simulink library "carnot"  (R2018b)
settings: Solver=VariableStepAuto  StartTime=0.0  StopTime=10.0  RelTol=1e-3
undefined symbols (not defined in the file or in its folder): A, A_earth, acol, Acol, ActPower1, ActPower2, ActPower3, Ad, Ad0, Ar, Au, Au0, Azimuth_Angle, B, Bd, Bd0, Br, Bu, Bu0, C, c1, c2, c3, c33, c4, c5, c6, CarnotCallbacks_Density, CarnotCallbacks_Enthalpy, CarnotCallbacks_Enthalpy2Temperature, CarnotCallbacks_Entropy, CarnotCallbacks_Evaporation_Enthalpy, CarnotCallbacks_GlobalMessageLevel, CarnotCallbacks_Grashof, CarnotCallbacks_Heat_Capacity, CarnotCallbacks_Kinematic_Viscosity, CarnotCallbacks_PMV_PPD, CarnotCallbacks_Prandtl, CarnotCallbacks_Saturation_Property, CarnotCallbacks_Saturation_Temperature, CarnotCallbacks_Saturation_Value_Water, CarnotCallbacks_Specific_Volume, CarnotCallbacks_Thermal_Conductivity, CarnotCallbacks_Vapour_Content, CarnotCallbacks_Vapour_Pressure, Cd, Cdl, Cr, Cu, Davies, Dd, DE_TRY2010_04_averageYear, delta_grd, density, DiameterLastPiece, dl, DPConstant, DPLinear, DPQuadratic, Dr ... (+59)
libraries: $bdroot x429, simulink x36, simulink_extras x12
(part 8 of 22)

== system carnot/Load/Houses ==
  House_simple : Subsystem  mask(House simple){tini=20, dtroom=inf, Tmeaninside=23.8, deltathetai=3.8, Tmeanoutside=11, deltathetae=9.3, tshift=319*3600, PathName=fullfile(path_carnot('libsl'), 'Load', 'Houses', 'House_simple', 'parameter_set'), FileName='Default_SimpleHouseISOgm.mat', userPath=off, userParam=off, Ahabit=140, Hroom=2.5, slabwidth=10, slablength=7, dwall=0.4, UAwall=100, capa=500000, utot=0.183, gammat=0, cond_ground=2, cp_ground=800, rho_ground=2500, Awindow=[12 4 3 4], AziWin=[0 90 -180 -90], Uwindow=[2 2 2 2], Gwindow=[0.5 0.5 0.5 0.5], alpha=10, H=1.2, W=1, Nwin=4, Ventilationrate=0.4, Heatrecovery=0, pnom=10000, dtnom=49.83, expo=1.3, mcap=10*4812, lin=100, qua=100}
      mask prompts: tini "Initial temperature in °C"; dtroom "Max. change of room temperature in K (standard value is 'inf')"; Tmeaninside "Mean inside temperature over one year [°C]"; deltathetai "Amplitude of monthly mean inside temperature over the year [K]"; Tmeanoutside "Mean outside temperature over one year [°C]"; deltathetae "Amplitude of monthly mean outside temperature over the year [K]"; tshift "Time shift where outside temperature sine-curve shows a mimimum [s]"; PathName "Path"; FileName "Parameter set"; userPath "Edit path and name of parameter set"; userParam "User defined parameters"; Ahabit "Heated living surface in m²"; Hroom "Height of rooms in m"; slabwidth "Width of slab in m"; slablength "Length of slab in m"; dwall "Average thickness of walls inlcuding insulation [m]"; UAwall "Total heat transfer to ambient (walls/roof) in W/K"; capa "Thermal capactiy per surface in J/m²/K"; utot "Total heat transfer of slab to ground [W/m²/K]"; gammat "linear thermal transmittance associated with wall/floor junctions [W/mK]"; cond_ground "conductivity of ground [W/(m*K)]"; cp_ground "capacity of ground [J/(kg*K)]"; rho_ground "density of ground [kg/m^3]"; Awindow "Surface of 4 windows in m² (vector)"; AziWin "Orientation of the 4 windows (south 0, east -90,west 90)"; Uwindow "Heat loss coefficient 4 windows in W/m²/K [vector]"; Gwindow "Light transmittance 4 windows (0..1) * (1 - frame_part) [vector]"; alpha "Maximal opening angle in °"; H "Height of window opening in m"; W "Width of window opening in m"; Nwin "Number of windows for ventilation"; Ventilationrate "Ventilation rate in 1/h"; Heatrecovery "Heat recovery (0..1)"; pnom "Qdot_nom: nominal power in W"; dtnom "Tdiff_nom: nominal temperature difference in K"; expo "Radiator exponent (> 0)"; mcap "mass * capacity in J/K"; lin "l : linear pressure drop Pa/(kg/s)"; qua "q : quadratic pressure drop Pa/(kg/s)²"
      mask help:
      | Simple model of a house with one thermal node. The geometry is a box with a flat roof and 4 windows (see House_OneNodeModel). The heat transfer to the ground is modeled by HeatTransfer2Ground_ISO13370. The heating system is the Radiator model. The ventilation an heat recovery uses the Ventilation model. Resident data like internal gains, window opening and shading are defined by the Resident Data Bus RDB.
      |
      | Max. change of room temperatue: Set parameter to 0 K to calculate idealized heating behaviour. The power balance (Qdot_all) is the theoretical heating demand (see example_House_Ideal.slx).
      mask init:
      | [ok, param] = CarnotCallbacks_HouseSimple('SetParameters',gcbh,PathName,FileName);
      mask Help: web(fullfile(path_carnot('help'),'houseSimple.html'),'-helpbrowser')
      mask TypeOptions tini: House_OneNodeModel/tini | Radiator/tini
      mask TypeOptions dtroom: House_OneNodeModel/dtroom
      mask TypeOptions Tmeaninside: HeatTransfer2Ground_ISO13370/Tmeaninside
      mask TypeOptions deltathetai: HeatTransfer2Ground_ISO13370/deltathetai
      mask TypeOptions Tmeanoutside: HeatTransfer2Ground_ISO13370/Tmeanoutside
      mask TypeOptions deltathetae: HeatTransfer2Ground_ISO13370/deltathetae
      mask TypeOptions tshift: HeatTransfer2Ground_ISO13370/tshift
      mask Callback userPath: [ok, param] = CarnotCallbacks_HouseSimple('UserEdit',gcbh);
      mask Callback userParam: [ok, param] = CarnotCallbacks_HouseSimple('UserEdit',gcbh);
      mask TypeOptions Ahabit: House_OneNodeModel/A | Ventilation/Ahabit | Ahabit/Value
      mask TypeOptions Hroom: Simple_House_ISO_GroundModel/Hroom | Ventilation/Hroom
      mask TypeOptions slabwidth: HeatTransfer2Ground_ISO13370/slabwidth
      mask TypeOptions slablength: HeatTransfer2Ground_ISO13370/slablength
      mask TypeOptions dwall: HeatTransfer2Ground_ISO13370/dwall
      mask TypeOptions UAwall: House_OneNodeModel/UAout
      mask TypeOptions capa: House_OneNodeModel/capa
      mask TypeOptions utot: HeatTransfer2Ground_ISO13370/utot
      mask TypeOptions gammat: HeatTransfer2Ground_ISO13370/gammat
      mask TypeOptions cond_ground: HeatTransfer2Ground_ISO13370/cond_ground
      mask TypeOptions cp_ground: HeatTransfer2Ground_ISO13370/cp_ground
      mask TypeOptions rho_ground: HeatTransfer2Ground_ISO13370/rho_ground
      mask TypeOptions Awindow: House_OneNodeModel/Awin
      mask TypeOptions AziWin: House_OneNodeModel/AziWin
      mask TypeOptions Uwindow: House_OneNodeModel/Uwin
      mask TypeOptions Gwindow: House_OneNodeModel/Gwin
      mask TypeOptions alpha: Ventilation/alpha
      mask TypeOptions H: Ventilation/H
      mask TypeOptions W: Ventilation/W
      mask TypeOptions Nwin: Ventilation/Nwin
      mask TypeOptions Ventilationrate: Ventilation/vent
      mask TypeOptions Heatrecovery: Ventilation/rec
      mask TypeOptions pnom: Radiator/pnom
      mask TypeOptions dtnom: Radiator/dtnom
      mask TypeOptions expo: Radiator/expo
      mask TypeOptions mcap: Radiator/mcap
      mask TypeOptions lin: Radiator/lin
      mask TypeOptions qua: Radiator/qua
      mask DialogControl Container10 Prompt: Calculation
      mask DialogControl ParameterGroupFile Prompt: Picking a parameter set
      mask DialogControl Control1 Prompt: Carnot public data
      mask DialogControl Control1 Callback: [ok, file] = CarnotCallbacks_HouseSimple('GetFilename',gcbh, 'public');
      mask DialogControl Control3 Prompt: Carnot internal data
      mask DialogControl Control3 Callback: [ok, file] = CarnotCallbacks_HouseSimple('GetFilename',gcbh, 'internal');
      mask DialogControl Control4 Prompt: Selected path
      mask DialogControl Control4 Callback: [ok, file] = CarnotCallbacks_HouseSimple('GetFilename',gcbh, 'selected');
      mask DialogControl Container5 Prompt: House
      mask DialogControl Container13 Prompt: Ground
      mask DialogControl Container8 Prompt: Windows
      mask DialogControl Container9 Prompt: HVAC
      mask DialogControl Control5 Prompt: Save in Carnot internal data
      mask DialogControl Control5 Callback: [ok, param] = CarnotCallbacks_HouseSimple('SaveFilename',gcbh, 'internal','SH');
      mask DialogControl Control6 Prompt: Save in selected path
      mask DialogControl Control6 Callback: [ok, param] = CarnotCallbacks_HouseSimple('SaveFilename',gcbh, 'selected','SH');
      mask Display:
      | % user defined picture file
      | picfile = fullfile(path_carnot('intlibsl'), ...
      |         'Load','Houses','Simple_House_ISOgm_CONF','parameter_set', ...
      |         'Simple_House_ISOgm_CONF.jpg');
      | 
      | % show internal picture if defined
      | if ~BlockIsInCarnotLibrary ...      % if not located in library any more
      |         && exist(picfile,'file')    % AND picfile is present
      |     image(imread(picfile), [0.15 0.1 0.7 0.8])
      |     set_param(gcb, 'BackgroundColor', 'White')
      | else
      |     % show public picture
      |     plot([10,10,90,90,10]/120+0.1, [0,50,50,0,0]/100+0.1,...
      |          [100,60,40,0]/120+0.1,    [40,80,80,40]/100+0.1,...
      |          [20,34,34,20,20]/120+0.1, [40,40,20,20,40]/100+0.1,...
      |          [60,60,40,40]/120+0.1,    [0,40,40,0]/100+0.1,...
      |          [65,80,80,65,65]/120+0.1, [40,40,20,20,40]/100+0.1,...
      |          [47,54,54,47,47]/120+0.1, [35,35,4,4,35]/100+0.1,...
      |          [45,41]/120+0.1,          [20,20]/100+0.1)
      |      set_param(gcb, 'BackgroundColor', 'Orange')
      | end
  Resident_Data : Subsystem  mask(Resident Task){CalcAirComp=on}
      mask prompts: CalcAirComp "Calculate the composition of room air (H2O, CO2, VOC)"
      mask help:
      | Create the Resident Data Bus.
      | Qdot_internal : internal gains in the building in W
      | Sunshade : shading of the windows [0..1]
      | 	0 : no shading
      | 	1 : complete shading
      | OpenWindow : open the windows [0..1]
      | 	0 : closed
      | 	1 : completely opened
      | Massflow_CO2 : massflow of CO2 generated by internal sources in kg/s
      | Massflow_H2O : massflow of HO generated by internal sources in kg/s
      | Massflow_VOC : massflow of VOCs generated by internal sources in kg/s
      mask TypeOptions CalcAirComp: CalculateAirComposition/CalcAirComp
      mask Display:
      | plot(-20,-20,100,100,[30,70,70,30,30],[80,80,30,30,80],...
      |     [65,60,40,35],[30,40,40,30],...
      |     [53,53,56,56,50,44,44,47,47],...
      |     [40,45,49,60,65,60,50,45,40],...
      |     [57,50,44],[40,34,40],...
      |     [52,53],[55,55],[47,48],[55,55],...
      |     [56,53,47,44],[51,60,60,51],[52,50,48],[49,48,49])
  Resident_Task44 : Subsystem  mask(Resident Task){period=24*3600, rep_seq_te=[0 1 6 7 8 9 11 12 13 18 19 20 22 23]*3600, rep_seq_de=[1 5 1 1 1 2 1 1 4 2 1 2 1 1]*3600, rep_seq_ye=[105 55 392.5 457.5 420 55 250 55 120 170 615 420 442.5 355], rep_seq_to=[0 6 7 8 9 11 12 13 14 15 17 18 20 21 22]*3600, rep_seq_do=[6 1 1 1 2 1 1 1 1 2 1 2 1 1 2]*3600, rep_seq_yo=[4 2 3 2 0 1 3 2 1 0 1 2 4 3 4]*60, Topen=24, Tclose=23, TrAboveTa=2, TaTooCold=12, timeFIR=24, TaIni=12, starttime=8, stoptime=22, TroomShadeOn=23.8, TroomShadeOff=22.8, SolarShadeOn=300, SolarShadeOff=200, max_shade=1, CalcAirComp=off, mdotCO2=0, mdotH2O=0, mdotVOC=0}
      mask prompts: period "Time period in s"; rep_seq_te "Time values in s"; rep_seq_de "Duration in s"; rep_seq_ye "Internal gains due to electricity consumption in W"; rep_seq_to "Time values in s"; rep_seq_do "Duration in s"; rep_seq_yo "Internal gain due to persons in W"; Topen "Open window if Troom is above [°C]"; Tclose "Close window if Troom is below [°C]"; TrAboveTa "Open window if Troom is above Tamb [K]"; TaTooCold "Close window if average Tamb is below [°C]"; timeFIR "Average time for Tamb in h (only integer values)"; TaIni "Initial value for Tamb in °C"; starttime "Start time in the morning [h]"; stoptime "Stop time in the evening [h]"; TroomShadeOn "Room temperature to switch shading on in °C"; TroomShadeOff "Room temperature to switch shading off in °C"; SolarShadeOn "Solar radiation to switch shading on in W/m²"; SolarShadeOff "Solar radiation to switch shading off in W/m²"; max_shade "Maximum value for Sunshade"; CalcAirComp "Calculate the composition of room air (H2O, CO2, VOC)"; mdotCO2 "Massflow CO2 in kg/s"; mdotH2O "Massflow H2O in kg/s"; mdotVOC "Massflow VOC in kg/s"
      mask help: Create the Resident Data Bus for boundary conditions of Task 44.
      mask TypeOptions period: Electric_Gains_Profile/period | Occupation_Profile/period
      mask TypeOptions rep_seq_te: Electric_Gains_Profile/rep_seq_t
      mask TypeOptions rep_seq_de: Electric_Gains_Profile/rep_seq_d
      mask TypeOptions rep_seq_ye: Electric_Gains_Profile/rep_seq_y
      mask TypeOptions rep_seq_to: Occupation_Profile/rep_seq_t
      mask TypeOptions rep_seq_do: Occupation_Profile/rep_seq_d
      mask TypeOptions rep_seq_yo: Occupation_Profile/rep_seq_y
      mask TypeOptions Topen: Window_Control/Topen
      mask TypeOptions Tclose: Window_Control/Tclose
      mask TypeOptions TrAboveTa: Window_Control/TrAboveTa
      mask TypeOptions TaTooCold: Window_Control/TaTooCold
      mask TypeOptions timeFIR: Window_Control/timeFIR
      mask TypeOptions TaIni: Window_Control/TaIni
      mask TypeOptions starttime: Window_Control/starttime
      mask TypeOptions stoptime: Window_Control/stoptime
      mask TypeOptions TroomShadeOn: Shading_Control/TroomShadeOn
      mask TypeOptions TroomShadeOff: Shading_Control/TroomShadeOff
      mask TypeOptions SolarShadeOn: Shading_Control/SolarShadeOn
      mask TypeOptions SolarShadeOff: Shading_Control/SolarShadeOff
      mask TypeOptions max_shade: Shading_Control/max_shade
      mask TypeOptions CalcAirComp: CalculateAirComposition/CalcAirComp
      mask TypeOptions mdotCO2: Massflow_CO2/Value
      mask TypeOptions mdotH2O: Massflow_H2O/Value
      mask TypeOptions mdotVOC: Massflow_VOC/Value
      mask DialogControl Container5 Prompt: Internal gain
      mask DialogControl Container6 Prompt: Electric gains profile
      mask DialogControl Container7 Prompt: Occupation profile
      mask DialogControl Container8 Prompt: Windows
      mask DialogControl Container10 Prompt: Ventilation cooling
      mask DialogControl Container9 Prompt: Shading
      mask DialogControl Container11 Prompt: Emissions
      mask Display:
      | plot(0,0,100,100,[30,70,70,30,30],[80,80,30,30,80],...
      |     [65,60,40,35],[30,40,40,30],...
      |     [53,53,56,56,50,44,44,47,47],...
      |     [40,45,49,60,65,60,50,45,40],...
      |     [57,50,44],[40,34,40],...
      |     [52,53],[55,55],[47,48],[55,55],...
      |     [56,53,47,44],[51,60,60,51],[52,50,48],[49,48,49])
      | disp('\n\n\n\n\nTASK 44')
  Room_Floor_Heating : Subsystem  mask(room){t0=20, temp_neighbour=20}
      mask prompts: t0 "start temperature of rooms in °C"; temp_neighbour "temperature of rooms above and below in °C"
      mask help:
      | The block models of a heat transfer characteristic of two neighbour rooms.
      | Use "look under mask" to set up the models parameters (initial conditions,
      | floors and wall characteristics...)
      mask init:
      | AIV_neighbour = [0 temp_neighbour temp_neighbour 0 0 0 0 0 0];
      | zonefloordist2grnd = 0;
      mask Help: web(fullfile(path_carnot('help'),'Room_Floor_Heating.html'),'-helpbrowser')
      mask Display: plot(0,0,100,100,[30,30,60,60,30],[20,50,50,20,20],[47,47,56,56,47],[40,30,30,40,40],[42,42,34,34],[20,40,40,20],[62,45,28],[48,70,48])
  Room_Radiator : Subsystem  mask(room){t0=20, temp_neighbour=20}
      mask prompts: t0 "start temperature of rooms in °C"; temp_neighbour "temperature of rooms above and below in °C"
      mask help:
      | The block models of a heat transfer characteristic of two neighbour rooms.
      | Use "look under mask" to set up the models parameters (initial conditions,
      | floors and wall characteristics...)
      mask init:
      | AIV_neighbour = [0 temp_neighbour temp_neighbour 0 0 0 0 0 0];
      | zonefloordist2grnd = 0;
      mask Help: web(fullfile(path_carnot('help'),'Room_Radiator.html'),'-helpbrowser')
      mask Display: plot(0,0,100,100,[30,30,60,60,30],[20,50,50,20,20],[47,47,56,56,47],[40,30,30,40,40],[42,42,34,34],[20,40,40,20],[62,45,28],[48,70,48])

== system carnot/Outputs/AIV_selector ==
  "[AIV]" : Inport
  Selector : Selector  InputPortWidth=9  IndexOptions=Index vector (dialog)  Indices=v  OutputSizes=1
  "[AIV]s" : Outport
  wires:
  Selector/1 -> "[AIV]s"/1
  "[AIV]"/1 -> Selector/1

== system carnot/Outputs/Display_THB1 ==
  THB_yellow : Inport
  Selector : Selector  InputPortWidth=20  IndexOptions=Index vector (dialog)  Indices=[v]  OutputSizes=1
  THB2THV : $bdroot/Toolbox/THB2THV
  to_scope : Outport
  wires:
  Selector/1 -> to_scope/1
  THB_yellow/1 -> THB2THV/1
  THB2THV/1 -> Selector/1

== system carnot/Outputs/Display_THB2 ==
  THB_yellow : Inport
  THB_blue : Inport  Port=2
  Mux : Mux  Inputs=2
  Selector : Selector  InputPortWidth=20  IndexOptions=Index vector (dialog)  Indices=[v]  OutputSizes=1
  Selector1 : Selector  InputPortWidth=20  IndexOptions=Index vector (dialog)  Indices=[v]  OutputSizes=1
  THB2THV1 : $bdroot/Toolbox/THB2THV
  THB2THV2 : $bdroot/Toolbox/THB2THV
  to_scope : Outport
  wires:
  THB_yellow/1 -> THB2THV1/1
  Selector/1 -> Mux/1
  THB_blue/1 -> THB2THV2/1
  Mux/1 -> to_scope/1
  Selector1/1 -> Mux/2
  THB2THV1/1 -> Selector/1
  THB2THV2/1 -> Selector1/1

== system carnot/Outputs/Display_THB3 ==
  THB_yellow : Inport
  THB_blue : Inport  Port=2
  THB_brown : Inport  Port=3
  Mux : Mux  Inputs=3
  Selector : Selector  InputPortWidth=20  IndexOptions=Index vector (dialog)  Indices=[v]  OutputSizes=1
  Selector1 : Selector  InputPortWidth=20  IndexOptions=Index vector (dialog)  Indices=[v]  OutputSizes=1
  Selector2 : Selector  InputPortWidth=20  IndexOptions=Index vector (dialog)  Indices=[v]  OutputSizes=1
  THB2THV1 : $bdroot/Toolbox/THB2THV
  THB2THV2 : $bdroot/Toolbox/THB2THV
  THB2THV3 : $bdroot/Toolbox/THB2THV
  to_scope : Outport
  wires:
  THB2THV3/1 -> Selector2/1
  THB2THV2/1 -> Selector1/1
  THB2THV1/1 -> Selector/1
  THB_yellow/1 -> THB2THV1/1
  Selector/1 -> Mux/1
  THB_blue/1 -> THB2THV2/1
  Mux/1 -> to_scope/1
  Selector1/1 -> Mux/2
  THB_brown/1 -> THB2THV3/1
  Selector2/1 -> Mux/3

== system carnot/Outputs/Display_THB4 ==
  THB_yellow : Inport
  THB_blue : Inport  Port=2
  THB_brown : Inport  Port=3
  THB_green : Inport  Port=4
  Mux : Mux
  Selector{,1..3} (4 alike) : Selector  InputPortWidth=20  IndexOptions=Index vector (dialog)  Indices=[v]  OutputSizes=1
  THB2THV{1..4} (4 alike) : $bdroot/Toolbox/THB2THV
  to_scope : Outport
  wires:
  Selector3/1 -> Mux/4
  THB_green/1 -> THB2THV4/1
  Selector2/1 -> Mux/3
  THB_brown/1 -> THB2THV3/1
  Selector1/1 -> Mux/2
  Mux/1 -> to_scope/1
  THB_blue/1 -> THB2THV2/1
  Selector/1 -> Mux/1
  THB_yellow/1 -> THB2THV1/1
  THB2THV1/1 -> Selector/1
  THB2THV2/1 -> Selector1/1
  THB2THV3/1 -> Selector2/1
  THB2THV4/1 -> Selector3/1

== system carnot/Outputs/Display_THB5 ==
  THB_yellow : Inport
  THB_magenta : Inport  Port=2
  THB_cyan : Inport  Port=3
  THB_red : Inport  Port=4
  THB_green : Inport  Port=5
  Mux : Mux  Inputs=5
  Selector{,1..4} (5 alike) : Selector  InputPortWidth=20  IndexOptions=Index vector (dialog)  Indices=[v]  OutputSizes=1
  THB2THV{1..5} (5 alike) : $bdroot/Toolbox/THB2THV
  to_scope : Outport
  wires:
  THB2THV5/1 -> Selector4/1
  THB2THV4/1 -> Selector3/1
  THB2THV3/1 -> Selector2/1
  THB2THV2/1 -> Selector1/1
  THB2THV1/1 -> Selector/1
  Mux/1 -> to_scope/1
  Selector/1 -> Mux/1
  THB_yellow/1 -> THB2THV1/1
  Selector1/1 -> Mux/2
  THB_magenta/1 -> THB2THV2/1
  Selector3/1 -> Mux/4
  THB_red/1 -> THB2THV4/1
  Selector2/1 -> Mux/3
  THB_cyan/1 -> THB2THV3/1
  THB_green/1 -> THB2THV5/1
  Selector4/1 -> Mux/5

== system carnot/Outputs/Display_THB6 ==
  THB_yellow : Inport
  THB_blue : Inport  Port=2
  THB_brown : Inport  Port=3
  THB_green : Inport  Port=4
  THB_purple : Inport  Port=5
  THB_cyan : Inport  Port=6
  Mux : Mux  Inputs=6
  Selector{,1..5} (6 alike) : Selector  InputPortWidth=20  IndexOptions=Index vector (dialog)  Indices=[v]  OutputSizes=1
  THB2THV{1..6} (6 alike) : $bdroot/Toolbox/THB2THV
  to_scope : Outport
  wires:
  THB_cyan/1 -> THB2THV6/1
  Selector5/1 -> Mux/6
  Selector4/1 -> Mux/5
  THB_purple/1 -> THB2THV5/1
  THB_brown/1 -> THB2THV3/1
  Selector2/1 -> Mux/3
  THB_green/1 -> THB2THV4/1
  Selector3/1 -> Mux/4
  THB_blue/1 -> THB2THV2/1
  Selector1/1 -> Mux/2
  THB_yellow/1 -> THB2THV1/1
  Selector/1 -> Mux/1
  Mux/1 -> to_scope/1
  THB2THV1/1 -> Selector/1
  THB2THV2/1 -> Selector1/1
  THB2THV3/1 -> Selector2/1
  THB2THV4/1 -> Selector3/1
  THB2THV5/1 -> Selector4/1
  THB2THV6/1 -> Selector5/1

== system carnot/Outputs/PMV_PPD ==
  LoadPerPerson : Inport
  MechanicalLoad : Inport  Port=2
  ClothingInsulation : Inport  Port=3
  AirTemperature : Inport  Port=4
  RadiationTemperature : Inport  Port=5
  AirVelocity : Inport  Port=6
  PartialPressureVapour : Inport  Port=7
  Terminator_ClothingAreaFactor : Terminator
  Terminator_HeatTransferCoefficient : Terminator
  comfortsfcn : S-Function  FunctionName=comfortsfcn  Parameters=DEBUGLEVEL-1, MAXTOTALWARNINGS, MAXCONSECUTIVEWARNINGS, WRITETOFILE, FILENAME  SFunctionDeploymentMode=off  EnableBusSupport=off
  PMV : Outport
  PPD : Outport  Port=2
  ClothingTemperature : Outport  Port=3
  wires:
  comfortsfcn/5 -> Terminator_HeatTransferCoefficient/1
  comfortsfcn/4 -> Terminator_ClothingAreaFactor/1
  comfortsfcn/3 -> ClothingTemperature/1
  comfortsfcn/2 -> PPD/1
  comfortsfcn/1 -> PMV/1
  AirVelocity/1 -> comfortsfcn/6
  RadiationTemperature/1 -> comfortsfcn/5
  ClothingInsulation/1 -> comfortsfcn/3
  MechanicalLoad/1 -> comfortsfcn/2
  LoadPerPerson/1 -> comfortsfcn/1
  AirTemperature/1 -> comfortsfcn/4
  PartialPressureVapour/1 -> comfortsfcn/7

== system carnot/Outputs/S_selector ==
  "[S]" : Inport
  Selector : Selector  InputPortWidth=13  IndexOptions=Index vector (dialog)  Indices=v  OutputSizes=1
  "[S]s" : Outport
  wires:
  "[S]"/1 -> Selector/1
  Selector/1 -> "[S]s"/1

== system carnot/Outputs/Sensitive_Room_Temperature ==
  note: Sensitive temperature
  "[AIV]" : Inport
  1-share_c : Gain  Gain=1-share_c  SaturateOnIntegerOverflow=on  OutDataTypeStr=Inherit: Same as input  ParamDataTypeStr=Inherit: Same as input
  Demux : Demux  Outputs=[1 1 1 6]
  Sum : Sum  SaturateOnIntegerOverflow=on  InputSameDT=on  OutDataTypeStr=Inherit: Same as first input
  Terminator1 : Terminator
  Terminator2 : Terminator
  share_c : Gain  Gain=share_c  SaturateOnIntegerOverflow=on  OutDataTypeStr=Inherit: Same as input  ParamDataTypeStr=Inherit: Same as input
  Ts : Outport
  wires:
  Demux/1 -> Terminator2/1
  Sum/1 -> Ts/1
  1-share_c/1 -> Sum/2  "Tr"
  share_c/1 -> Sum/1  "Tc"
  Demux/4 -> Terminator1/1
  "[AIV]"/1 -> Demux/1
  Demux/2 -> share_c/1
  Demux/3 -> 1-share_c/1

== system carnot/Outputs/THV_select ==
  THV : Inport
  Selector : Selector  InputPortWidth=20  IndexOptions=Index vector (dialog)  Indices=[v]  OutputSizes=1
  out : Outport  InitialOutput=0
  wires:
  Selector/1 -> out/1
  THV/1 -> Selector/1

== system carnot/Outputs/display_weather ==
  weather : Inport
  select_weather : $bdroot/Weather/Select_Weather  v=v
  to scope : Outport
  wires:
  select_weather/1 -> to scope/1
  weather/1 -> select_weather/1

== system carnot/Source/Boiler ==
  Condensing_Boiler : Subsystem  mask(Condensing Boiler){Tini=20, PathName=fullfile(path_carnot('libsl'), 'Source', 'Boiler', 'Condensing_Boiler', 'parameter_set'), FileName='CondensingBoiler_20kW.mat', userPath=off, userParam=off, Pgas=20000, HeatLoss=2.5, Volume=0.0035, whichTforEfficiency=mean of inlet and outlet temperature, TableRelativePower=[0 0.1 1], TableTemperatures=[10 50 90], TableData=[1 1 1; 1.08 0.92 0.85; 1.06 0.9 0.83], ElectricPower=[0 50 200], relQdotMin=0.1, dplin=10, dpqua=100, nodes=3}
      mask prompts: Tini "Initial temperature in °C"; PathName "Path"; FileName "Parameter set"; userPath "Edit path and name of parameter set"; userParam "User defined parameters"; Pgas "Heat input (= hi * GasMassflow) [W]"; HeatLoss "Heat losses in W/K"; Volume "Volume (of water) in m³"; whichTforEfficiency "Efficiency based on :"; TableRelativePower "Relative power in 0..1 : Breakpoints for electric power table and rows of efficiency table"; TableTemperatures "Temperature in °C : Breakpoints for columns in efficiency table"; TableData "Efficiency (Matrix) : rows for relative power, columns for temperature"; ElectricPower "Electric power in W (vector, one value for each value of the relative power)"; relQdotMin "Minimum control signal for "ON""; dplin "l : linear pressure drop Pa/(kg/s)"; dpqua "q : quadratic pressure drop Pa/(kg/s)²"; nodes "Number of thermal nodes"
      mask help: Multinode one-dimensional model of a boiler. Condensing effects are taken in account by an efficiency lookup table.
      mask init:
      | % callback to set parameters of model
      | [ok, param] = CarnotCallbacks_CondensingBoilerConf('SetParameters',gcbh,PathName,FileName);
      mask Help: web(fullfile(path_carnot('help'),'Condensing_Boiler.html'),'-helpbrowser')
      mask TypeOptions Tini: sfunBoiler/Tini
      mask Callback userPath: [ok, param] = CarnotCallbacks_CondensingBoilerConf('UserEdit',gcbh);
      mask Callback userParam: [ok, param] = CarnotCallbacks_CondensingBoilerConf('UserEdit',gcbh);
      mask TypeOptions Pgas: Pgas/Gain
      mask TypeOptions HeatLoss: sfunBoiler/UA
      mask TypeOptions Volume: sfunBoiler/vol
      mask TypeOptions whichTforEfficiency: SelectTefficiency/whichTforEfficiency
      mask TypeOptions TableRelativePower: TableEfficiency/BreakpointsForDimension1 | TablePelec/BreakpointsForDimension1
      mask TypeOptions TableTemperatures: TableEfficiency/BreakpointsForDimension2
      mask TypeOptions TableData: TableEfficiency/Table
      mask TypeOptions ElectricPower: TablePelec/Table
      mask TypeOptions relQdotMin: limitCtrl/relQdotMin
      mask TypeOptions dplin: Pressure_Drop_Fix/lin
      mask TypeOptions dpqua: Pressure_Drop_Fix/qua
      mask TypeOptions nodes: sfunBoiler/nodes
      mask DialogControl ParameterGroupFile Prompt: Picking a parameter set
      mask DialogControl Control1 Prompt: Carnot public data
      mask DialogControl Control1 Callback: [ok, file] = CarnotCallbacks_CondensingBoilerConf('GetFilename',gcbh,'public');
      mask DialogControl Control3 Prompt: Carnot internal data
      mask DialogControl Control3 Callback: [ok, file] = CarnotCallbacks_CondensingBoilerConf('GetFilename',gcbh,'internal');
      mask DialogControl Control4 Prompt: Selected path
      mask DialogControl Control4 Callback: [ok, file] = CarnotCallbacks_CondensingBoilerConf('GetFilename',gcbh,'selected');
      mask DialogControl PrameterGroupUser Prompt: Parameter Values
      mask DialogControl Container7 Prompt: Thermal
      mask DialogControl Container8 Prompt: Efficiency
      mask DialogControl Container9 Prompt: Hydraulic
      mask DialogControl Control7 Prompt: Pressure drop is: dp = l * mdot + q * mdot²
      mask DialogControl Container10 Prompt: Calculation
      mask DialogControl Control5 Prompt: Save in Carnot internal data
      mask DialogControl Control5 Callback: [ok, param] = CarnotCallbacks_CondensingBoilerConf('SaveFilename',gcbh,'internal','B');
      mask DialogControl Control6 Prompt: Save in selected path
      mask DialogControl Control6 Callback: [ok, param] = CarnotCallbacks_CondensingBoilerConf('SaveFilename',gcbh,'selected','B');
      mask Display:
      | % user defined picture file
      | picfile = fullfile(path_carnot('intlibsl'), ...
      |         'Source','Boiler','Condensing_Boiler','parameter_set', ...
      |         'Condensing_Boiler.jpg');
      | 
      | pic = false;
      | if ~BlockIsInCarnotLibrary    % if not located in library any more
      |     if exist(picfile,'file') % show internal picture if defined
      |         image(imread(picfile), [0.2, 0, 0.6, 1])
      |         set_param(gcb, 'BackgroundColor', 'White')
      |         pic = true;
      |     end
      | end
      | if ~pic    % show public picture
      |     set_param(gcb, 'BackgroundColor', 'Red')
      |     plot(0,0,1,1,[10,90,90,10,10]/100,[10,10,20,20,10]/100,[80,80,20,20]/100, ...
      |         [20,90,90,20]/100,[20,70,70,20]/100,[24,24,30,30]/100,[32,30,28]/100, ...
      |         [30,40,30]/100,[43,40,38]/100,[30,40,30]/100,[53,50,47]/100, ...
      |         [30,40,30]/100,[63,60,57]/100,[30,40,30]/100, ...
      |         [35,32,30,29,31,36,39,40,37,35]/100,[75,69,65,58,50,49,53,59,68,75]/100, ...
      |         [57,54,51,51,53,58,62,62,59,57]/100,[76,71,67,58,49,48,54,60,69,76]/100)
      | end
  Electric_Heater : Subsystem  mask(Electric Heater){}
      mask help: Heats the mass flow defined by the thermo-hydraulic bus with an electric power [W] entering the block.
      mask Help: web(fullfile(path_carnot('help'),'electric_heating.html'),'-helpbrowser')
      mask Display:
      | plot(0,0,100,100,[50,50,60,40,50],[55,40,70,60,90],[59,50],[48,40])
      | port_label('input',1,'THB')
      | port_label('input',2,'Qdot')
      | port_label('output',1,'THB')
  Electric_Heater_Ctrl : Subsystem  mask(Electric Heater Ctrl){power=1000, UA=1, mcp=3*4182}
      mask prompts: power "Electric heating power in W"; UA "UA: thermal loss coefficient in W/K"; mcp "mcp: thermal capacity of the node in J/K"
      mask help:
      | Heats the mass flow defined in the thermo-hydraulic bus with an electric power [W]. The model has a thermal interia (Thermal Node) and losses to the ambient. The initial temperature of the thermal node is the ambient temperature.
      | mcp * dT/dt = UA*(Tamb-T) + mdot*cp_in*(Tin-T)
      |                       + Ctrl*Electric_heating_power
      | cp_in  :  heat capacity of entering fluid in J/kg/K
      | Ctrl  :  Control input, range [0...1]
      | mdot  :  entering fluid massflow in kg/s
      | Tamb : ambient temperature input in °C (for thermal losses)
      | Tin   :  temperature of entering massflow in °C
      | T     :  temperature of the node and outlet in °C
      mask Help: web(fullfile(path_carnot('help'),'Electric_Heater_Ctrl.html'),'-helpbrowser')
      mask TypeOptions power: Gain/Gain
      mask TypeOptions UA: Thermal_Node/UA
      mask TypeOptions mcp: Thermal_Node/mcp
      mask Display: plot(0,0,100,100,[50,50,60,40,50],[55,40,70,60,90],[59,50],[48,40])

== system carnot/Source/Chiller ==
  Absorption_Chiller_LookUp : Subsystem  LoadFcn=|  mask(Absorption_Chiller_LookUp){chillertype=Yazaki WFC-SC5, heating_T_heating=[70 71 72 73 74 75 76 77 78 79 80 81 82 83 84 85 86 87 88], heating_T_recooling=[29 31 33], heating_T_cooling=[11 12.5 14], heating_Qdot=1000*cat(3, [11.5881 9.1729 7.1257; 12.7010 10.3602 8.4661; 13.7629 11.4453 9.5786; 14.7846 12.4541 10.5382; 15.7779 13.4104 11.3994; 16.7568 14.3365 12.1994; 17.7369 15.2538 12.9661; 18.7352 16.1871 13.7316; 19.7725 17.1783 14.5620; 20.8727 18.2790 15.5386; 21.4613 18.7997 16.0051; 22.1221 19.4526 16.6571; 22.8301 20.1885 17.4171; 23.5620 20.9610 18.2116; 24.3132 21.7625 19.0310; 25.0838 22.5963 19.8849; 25.8734 23.4650 20.7822; 26.6798 24.3672 21.7227; 27.5000 25.3000 22.7026], [11.5770 9.1404 7.0019; 12.7946 10.4820 8.5464; 13.9519 11.6809 9.7954; 15.0589 12.7736 10.8503; 16.1256 13.7910 11.7810; 17.1622 14.7571 12.6313; 18.1791 15.6924 13.4319; 19.1897 16.6217 14.2164; 20.2208 17.5967 15.0560; 21.3053 18.6810 16.0354; 21.9686 19.2406 16.5703; 22.7017 19.9403 17.2856; 23.4728 20.7187 18.0972; 24.2533 21.5195 18.9268; 25.0400 22.3359 19.7666; 25.8372 23.1759 20.6298; 26.6482 24.0459 21.5289; 27.4705 24.9436 22.4620; 28.3000 25.8635 23.4225], [11.6060 9.2707 7.0732; 12.8444 10.5919 8.6463; 14.0314 11.8008 9.9499; 15.1740 12.9258 11.0711; 16.2788 13.9911 12.0715; 17.3504 15.0094 12.9866; 18.3927 15.9884 13.8393; 19.4114 16.9403 14.6560; 20.4215 17.9043 15.5008; 21.4421 18.9298 16.4494; 22.3770 19.7105 17.1376; 23.3307 20.5777 17.9644; 24.2859 21.4864 18.8566; 25.2275 22.3953 19.7465; 26.1572 23.3020 20.6298; 27.0823 24.2153 21.5215; 28.0081 25.1426 22.4350; 28.9326 26.0813 23.3675; 29.8510 27.0252 24.3106]), recooling_T_heating=[70 79 88], recooling_T_recooling=[29 31 33], recooling_T_cooling=[11 12.5 14], recooling_Qdot=1000*cat(3, [17.7490 12.9282 8.7004; 34.7262 30.2580 25.0504; 45.9087 40.8416 35.7528], [17.2271 12.0716 8.2439; 35.4258 31.2730 26.0419; 48.6320 43.2955 38.4385], [17.2978 12.4414 8.1943; 35.0711 30.8160 26.3417; 52.3435 45.8810 40.5337]), cooling_T_heating=[70 79 88], cooling_T_recooling=[29 31 33], cooling_T_cooling=[11 12.5 14], cooling_Qdot=1000*cat(3, [7.0144 4.7740 2.6867; 14.9294 12.8469 10.4033; 19.0103 16.2646 13.7101], [6.8604 4.4520 2.5150; 15.2614 13.2863 10.9945; 20.4077 17.6879 15.3832], [6.9061 4.7080 2.6441; 15.1135 13.2179 11.1459; 22.6100 19.5272 17.0154]), deadtime_factor=11768, deadtime_exponent=-1.205}
      | load('THB.mat');
      | CarnotCallbacks_Absorption_Chiller_LookUp('CreateMaskStyles', gcb);
      | CarnotCallbacks_Absorption_Chiller_LookUp('CreateMaskVisibilities', gcb);
      mask prompts: chillertype "chiller type"; heating_T_heating "T heating beakpoints"; heating_T_recooling "T recooling beakpoints"; heating_T_cooling "T cooling beakpoints"; heating_Qdot "Q generator table"; recooling_T_heating "T heating beakpoints"; recooling_T_recooling "T recooling beakpoints"; recooling_T_cooling "T cooling beakpoints"; recooling_Qdot "Q recooling table"; cooling_T_heating "T heating beakpoints"; cooling_T_recooling "T recooling beakpoints"; cooling_T_cooling "T cooling beakpoints"; cooling_Qdot "Q cooling table"; deadtime_factor "factor"; deadtime_exponent "exponent"
      mask help: This block calculates the capacities and cop of an absorption chiller via a lookup table.
      mask init:
      | data = CarnotCallbacks_Absorption_Chiller_LookUp('GetChillerData', chillertype, heating_T_heating, heating_T_recooling, heating_T_cooling, heating_Qdot, recooling_T_heating, recooling_T_recooling, recooling_T_cooling, recooling_Qdot, cooling_T_heating, cooling_T_recooling, cooling_T_cooling, cooling_Qdot, deadtime_factor, deadtime_exponent);
      settings: AttributesFormatString=%<chillertype>
      mask Help: web(fullfile(path_carnot('help'),'absorption_chiller_lookup.html'),'-helpbrowser')
      mask TypeOptions chillertype: Yazaki WFC-SC5 | own data
      mask Callback chillertype: CarnotCallbacks_Absorption_Chiller_LookUp('CreateMaskVisibilities', gcb);
      mask DialogControl Container7 Prompt: chiller
      mask DialogControl Container4 Prompt: heating
      mask DialogControl Container9 Prompt: recooling
      mask DialogControl Container10 Prompt: cooling
      mask DialogControl Container11 Prompt: dead time
      mask Display: disp('Absorption\nChiller\nLookUp')
  Absorption_Chiller_ddT : Subsystem  mask(Absorption chiller model){E=1.2, sE=0.42, rE=0.9, sG=0.51, rG=2/0.51, dpe=[100 1e4], dpg=[100 1e4], Pel_p=80}
      mask prompts: E "E (A = 1+E)"; sE "s_e"; rE "r_e"; sG "s_g"; rG "r_g"; dpe "[linear quadratic] massflow dependant pressure drop evaporator in [Pa]"; dpg "[linear quadratic] massflow dependant pressure drop generator in [Pa]"; Pel_p "Pel solution pump [W]"
      mask help:
      | Empirical model of an absorption chiller based on the fitted deltadelta_t'
      | model from A. Kühn (2005) :
      |
      | Linear model:
      |  deltadelta_t'=t_G - A*t_AC + E*t_E
      |  Qdot_E = s_e * deltadelta_t' + r_e
      |  Qdot_G = s_g * deltadelta_t' + r_g
      |
      | Use acm_param.m to determine A, E, s_e, r_e, s_g and r_g with
      | characterisitics of the absorption chiller.
      mask Help: web(fullfile(path_carnot('help'),'absorption_chiller_ddt.html'),'-helpbrowser')
      mask Display: disp('Absorption\nChiller\nDeltaDeltaT\nModel')
  Compression_Air_Water_Chiller : Subsystem  mask(compression air/water chiller){Q_Nom=15}
      mask prompts: Q_Nom "Q_Nom [kW]"
      mask help:
      | This block is based on the characteristic curves for cooling capacity and
      | coefficient of performance of the reversible air-to-water heat pump with waste heat recovery LI 16TER+ by Dimplex.
      | The cooling capacity, coefficient of performance, electrical power and THV_WATER_OUT are calculated.
      | The air THV is not calculated due to missing interest.
      | The scaling is based on the point of 11.9 kW.
      |
      | Enter the cooling capacity for the point
      | T_AIR_IN= 30°C, T_WATER_OUT= 7°C.
      | A capacity between 5..50 kW is recommended.
      mask Help: web(fullfile(path_carnot('help'),'compression_chiller.html'),'-helpbrowser')
  Cooling_Tower : Subsystem  mask(Closed Circuit Cooling Tower){}
      mask help:
      | performance data
      | wet-bulb temperature - 15°C ... 24°C
      | rpm fan - 248 1/min (30%) ... 824 1/min (100%)
      | fluid temperature - 26°C ... 44°C
      | fluid flow rate - 1,07 l/s ... 3,03 l/s
      | water/glykol - 0 % ... 100%
      |
      | data logging:
      | wet-bulb temperature....[°C]   (ambient air)
      | rpm fan.........................[%]
      | v_dot fan......................[m³/s]
      | rpm fan.........................[1/min]
      | rel_hum.........................[%]     (ambient air)
      | t_air..............................[°C]    (ambient air)
      | energy ct......................[kJ]    (fan motor + recirculating spray pump)
      | power ct.......................[kW]    (fan motor + recirculating spray pump)
      | water consumption.......[kg]
      | Tnodes.........................[°C]    (inactivity modul)
      | THBout
      mask Help: web(fullfile(path_carnot('help'),'Cooling_Tower.html'),'-helpbrowser')
      mask Display:
      | plot(-20,5,140,80,[20 90 90 20 20],[20 20 70 70 20])
      | plot([30 35],[62 65],[40 35],[62 65],[35 35],[62 65],[80 80],[62 65],[75 80],[62 65],[85 80],[62 65],[57 57],[62 65],[52 57],[62 65],[62 57],[62 65])
      | plot([15 20],[22 22],[15 80],[65 65],[15 15],[22 65],[20 90],[24 24])
      | plot([25 100],[58 58],[25 100],[44 44],[60 25],[51 58],[60 25],[51 44])
      | plot([87 93],[36 36],[87 93],[28 28],[87 82],[36 34],[93 98],[36 34],[87 82],[28 30],[93 98],[28 30],[82 82],[34 30],[98 98],[34 30],[82 95],[34 35],[82 95],[30 29])
      | plot([86 90],[32 32],[90 93],[32 33.5],[90 93],[32 30.5])

== system carnot/Source/Cogeneration ==
  microCHP_constant : Subsystem  mask{P_th=11520, P_el=5500, P_fuel=22030, T_flow_setpoint=80, T_return_max=75}
      mask prompts: P_th "Nominal heating power [W] - at T_flow_out of 60°C"; P_el "Electrical power [W]"; P_fuel "Fuel power [W]"; T_flow_setpoint "T_flow_setpoint [°C] - Setpoint temperature of thermostat"; T_return_max "T_return_max [°C] - safety shutdown temperature"
      mask help:
      | This block is based on characteristic curves calculating heating capacity and representing a thermostat-controlled three-way mixer valve situated in the inlet flow of a gas driven micro-CHP called "Dachs" by Senertec. External mass flow rate, outlet flow temperature and heating power factor depend on inlet return temperature and are calculated by 1-D lookup-tables based on measured data.
      | The scaling is based on a heating power of 12.52 kW, an electrical power of 5.5 kW, a fuel power of 22,03 kW and a maximum external mass flow rate of 0.14 kg/s.
      | Mass flow rate and thermal inertia are linearly resized according to the inputed nominal heating power.
      mask Help: eval('filetest (''manual.htm#electric_heating'')')
      mask Display: plot(0,0,100,100,[50,50,60,40,50],[55,40,70,60,90],[59,50],[48,40])
  microCHP_modulating : Subsystem  mask(CHP){P_th_max=12500, P_th_min=3500, P_th_start=8000, f_P_el=0.37, T_flow_setpoint=80, T_flow_max=88, t_start=180, t_readjustment=450}
      mask prompts: P_th_max "maximum heating power [W]"; P_th_min "minimum heating power [W]"; P_th_start "initial heating power at start-up phase [W]"; f_P_el "electrical power fraction (referring to heating power) [0..1]"; T_flow_setpoint "flow setpoint temperature [°C]"; T_flow_max "maximum flow temperature [°C]"; t_start "duration of start-up phase [s]"; t_readjustment "duration of readjustment intervall [s]"
      mask help:
      | engine speed = f(T_return_load, T_flow_setpoint, T_flow, T_return)
      | T_return_load: a storage temperature or the return flow temperature.
      | Adjustable start-up phase: initial heating power
      | Ramp-up phase: maximum heating power up to 60°C
      | Control phase: heating power is readjusted after an inputed readjustment intervall.
      |
      | Return temperature raising facility.
      mask Help: eval('filetest (''manual.htm#electric_heating'')')
      mask Display: plot(0,0,100,100,[50,50,60,40,50],[55,40,70,60,90],[59,50],[48,40])

== system carnot/Source/Electric_Generator ==
  Inverter : Subsystem  mask(Inverter){PathName=fullfile(path_carnot('libsl'), 'Source', 'Electric_Generator', 'Inverter', 'parameter_set'), FileName='SMA_SB1_5_VL40.mat', userPath=off, userParam=off, Pacnom=1500, nphase=1-phase, U=230, f=50, PstepsEta=[0 0.1 0.2 0.25 0.3 0.5 0.75 1], Eta=[0 0.927 0.955 0.96 0.964 0.97 0.972 0.972], P_standby=1}
      mask prompts: PathName "Path"; FileName "Parameter set"; userPath "Edit path and name of parameter set"; userParam "User defined parameters"; Pacnom "Maximum AC power in W"; nphase "Number of phases"; U "Voltage of grid"; f "Frequency of grid"; PstepsEta "Breakpoints for efficiency (0..1)"; Eta "Efficiency table data (0..1)"; P_standby "Standby power in W"
      mask help: Model of an inverter e.g. for PV generators. The block considers the eficiency of the inverter in a lookup table.
      mask init:
      | % callback to set parameters of model
      | [ok, param] = CarnotCallbacks_InverterConf('SetParameters',gcbh,PathName,FileName);
      mask Help: web(fullfile(path_carnot('help'),'Inverter.html'),'-helpbrowser')
      mask Callback userPath: [ok, param] = CarnotCallbacks_InverterConf('UserEdit',gcbh);
      mask Callback userParam: [ok, param] = CarnotCallbacks_InverterConf('UserEdit',gcbh);
      mask TypeOptions Pacnom: NormialPower/Value | limit_Pacnom/UpperLimit
      mask TypeOptions nphase: Nphase/nphase
      mask TypeOptions U: Voltage/Value
      mask TypeOptions f: Frequency/Value
      mask TypeOptions PstepsEta: 1-D Lookup Table/BreakpointsForDimension1
      mask TypeOptions Eta: 1-D Lookup Table/Table
      mask TypeOptions P_standby: P_standby/Value
      mask DialogControl ParameterGroupFile Prompt: Picking a parameter set
      mask DialogControl Control2 Prompt: Carnot public data
      mask DialogControl Control2 Callback: [ok, file] = CarnotCallbacks_InverterConf('GetFilename',gcbh,'public');
      mask DialogControl Control3 Prompt: Carnot internal data
      mask DialogControl Control3 Callback: [ok, file] = CarnotCallbacks_InverterConf('GetFilename',gcbh,'internal');
      mask DialogControl Control4 Prompt: Selected path
      mask DialogControl Control4 Callback: [ok, file] = CarnotCallbacks_InverterConf('GetFilename',gcbh,'selected');
      mask DialogControl Control5 Prompt: Save in Carnot internal data
      mask DialogControl Control5 Callback: [ok, param] = CarnotCallbacks_InverterConf('SaveFilename',gcbh,'internal','IVRT');
      mask DialogControl Control6 Prompt: Save in selected path
      mask DialogControl Control6 Callback: [ok, param] = CarnotCallbacks_InverterConf('SaveFilename',gcbh,'selected','IVRT');
      mask Display:
      | pic = false;
      | if ~BlockIsInCarnotLibrary    % if not located in library any more
      |     picfile = fullfile(path_carnot('intlibsl'), ...
      |         'Source','Electric_Generator','Inverter','parameter_set', ...
      |         'Inverter.jpg');
      |     if exist(picfile,'file') % show internal picture if defined
      |         image(imread(picfile), [0.2, 0, 0.6, 1])
      |         set_param(gcb, 'BackgroundColor', 'White')
      |         pic = true;
      |     end
      | end
      | if ~pic    % show public picture
      |     set_param(gcb, 'BackgroundColor', 'Orange')
      |     plot(-40,0,140,100,...
      |         [90,10,90,90,10,10],[10,90,90,10,10,90],...
      |         [40,20],[40,40],[40,20],[30,30],...
      |         [88,84,75,64,55,50],[70,60,60,80,80,70])
      | end
  Inverter_SPI : Subsystem  mask(Inverter_SPI){PathName=fullfile(path_carnot('libsl'), 'Source', 'Electric_Generator', 'Inverter_SPI', 'parameter_set'), FileName='Kostal_Plenticicore_5p5_BatterBox_H11p5.mat', userPath=off, userParam=off, nphase=3-phase, soc0=soc0, socMin=socMin, socMax=socMax, Tsample=Tstest, capUser=0, SpiData=[5.686;5.487;6.35626283367556;6.191;5.419;0;73.4437227313543;94.5955883042527;31.1212070123701;74.9053455860837;92.4754002317794;31.7469866284786;30.8769273130404;90.5542640263268;41.6993897221684;86.4449570278825;105.13781756438;31.4770198650726;1;1;1;1;1;1;0.98;0.98;1.32333333333333;0.15;0;4.47;4.56;1.55;10.7670579897002;95.2833]}
      mask prompts: PathName "Path"; FileName "Parameter set"; userPath "Edit path and name of parameter set"; userParam "User defined parameters"; nphase "Number of phases"; soc0 "Initial State of Charge (0..1)"; socMin "Min. State of Charge (0..1)"; socMax "Max. State of Charge (0..1)"; Tsample "Sample Time (default =1s) [s]"; capUser "Battery capacity  (<=0 for default) [kWh]"; SpiData "SPI Parameter Set"
      mask help:
      | Hybrid Inverter with DC Battery
      | Efficiency of all power pahts is calculated by quadratic loss equation. Simple control dynamics are implemented as PT1 behavior.
      | This model is a simulink conversion of PermodDC Model by HTW Berlin.
      mask init:
      | % callback to set parameters of model
      | [ok, param] = CarnotCallbacks_Inverter_SPI('SetParameters',gcbh,PathName,FileName);
      mask Help: web(fullfile(path_carnot('help'),'Inverter_SPI.html'),'-helpbrowser')
      mask Callback userPath: [ok, param] = CarnotCallbacks_Inverter_SPI('UserEdit',gcbh);
      mask Callback userParam: [ok, param] = CarnotCallbacks_Inverter_SPI('UserEdit',gcbh);
      mask TypeOptions nphase: Nphase/nphase
      mask TypeOptions soc0: S-Function/soc0
      mask TypeOptions socMin: S-Function/soc_min
      mask TypeOptions socMax: S-Function/soc_max
      mask TypeOptions Tsample: S-Function/inv_Ts
      mask TypeOptions capUser: S-Function/cap_user
      mask TypeOptions SpiData: S-Function/spi_data
      mask DialogControl ParameterGroupFile Prompt: Picking a parameter set
      mask DialogControl Control2 Prompt: Carnot public data
      mask DialogControl Control2 Callback: [ok, file] = CarnotCallbacks_Inverter_SPI('GetFilename',gcbh,'public');
      mask DialogControl Control3 Prompt: Carnot internal data
      mask DialogControl Control3 Callback: [ok, file] = CarnotCallbacks_Inverter_SPI('GetFilename',gcbh,'internal');
      mask DialogControl Control4 Prompt: Selected path
      mask DialogControl Control4 Callback: [ok, file] = CarnotCallbacks_Inverter_SPI('GetFilename',gcbh,'selected');
      mask DialogControl Container7 Prompt: Parameters
      mask Display:
      | pic = false;
      | if ~BlockIsInCarnotLibrary    % if not located in library any more
      |     picfile = fullfile(path_carnot('intlibsl'), ...
      |         'Source','Electric_Generator','Inverter_SPI','parameter_set', ...
      |         'Inverter_SPI.jpg');
      |     if exist(picfile,'file') % show internal picture if defined
      |         image(imread(picfile), [0.2, 0, 0.6, 1])
      |         set_param(gcb, 'BackgroundColor', 'White')
      |         pic = true;
      |     end
      | end
      | if ~pic    % show public picture
      |     set_param(gcb, 'BackgroundColor', 'Orange')
      |     xo=0;
      |     plot(0,0,100,100,...
      |         xo+[76,30,76,76,30,30],[45,95,95,45,45,95],...
      |         xo+[35,45],[60,60],[35,45],[55,55],...
      |         xo+[73,71,67,63,59,57],[80,75,75,85,85,80],...
      |         xo+[76,30,30,76,76],[5,5,35,35,5],...)
      |         [53,53],[35,45],[55,55],[35,45],...
      |         [38.5,41.5],[30,30],[40,40],[28,32],xo+[64,68],[30,30])
      | end
  PV_Generator : Subsystem  mask(PV_Module_simple){Wp=5000, delta_Wp_K=0.0047, fgen=0.91 % 0.06 power missmatch, 0.01 diodes, 0.02 data sheet tolerance}
      mask prompts: Wp "Peak power of the generator [W]"; delta_Wp_K "Temperature coefficient Pmax 1/K"; fgen "efficiency generator field (lossses in diodes, power missmatch, dirt)"
      mask help:
      | This block simultes a PV module or generatater and calculates the DC power based on the parameters:
      | - Wp of one module or generator at STC [W]
      | - temperature coefficient of Pmax [1/K]
      | - dirt and degradation effects
      | The output DC power of the PV generator is ActPower1 in EB (power only)
      mask Help: web(fullfile(path_carnot('help'),'PV_Generator.html'),'-helpbrowser')
      mask Display: plot(0,0,100,100,[10,40,90,60,10],[10,90,90,10,10],[37,53,60,43,37],[70,70,86,86,70],[60,75,82,67,60],[70,71,86,86,70],[35,30,43,51,35],[65,50,49,65,65],[51,67,73,58,51],[50,50,66,66,50],[28,20,36,43,28],[41,23,23,41,41],[49,44,58,65,49],[41,23,22,41,41])
